simulink model "nonlinsim_bonus"  (R2025a)
settings: Solver=FixedStepAuto  StartTime=0.0  StopTime=100  FixedStep=0.01  RelTol=1e-3
values from neighbouring files (symbols this model uses):
  K_full = zeros(3, 12)    [FP_P9.m]
  u1o = (M + m) * g    (= 5659.275)    [FP_P9.m]    (also in nonlinsim_script.m)
  u2o = 0    [FP_P9.m]    (also in nonlinsim_script.m)
  u3o = 0    [FP_P9.m]    (also in nonlinsim_script.m)
settings Model: Creator=jonl6  LastModifiedBy=kritt
settings SolverCC: AlgebraicLoopSolver=TrustRegion
settings DebuggingCC: UnconnectedInputMsg=warning  UnconnectedOutputMsg=warning  UnconnectedLineMsg=warning
settings ModelReferenceCC: EnableRefExpFcnMdlSchedulingChecks=on
settings RTWCC: GPUComputeCapability=3.5

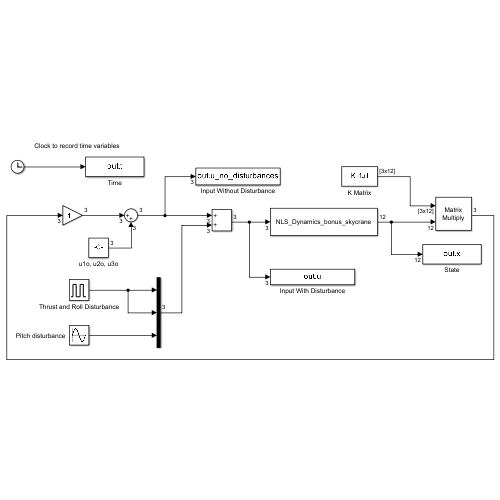
[thumbnail: Simulink's stored preview of the top-level diagram]
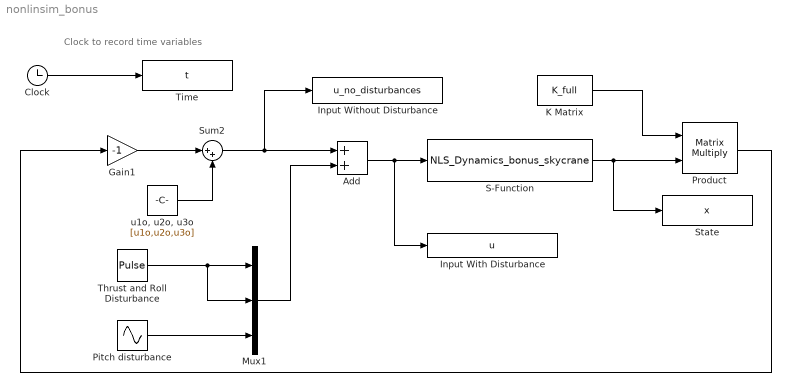
== system nonlinsim_bonus ==
  note: Clock to record time variables
  Add : Sum
  Clock : Clock
  Gain1 : Gain  Gain=-1
  Input With Disturbance : ToWorkspace  VariableName=u  SampleTime=-1
  Input Without Disturbance : ToWorkspace  VariableName=u_no_disturbances  SampleTime=-1
  K Matrix : Constant  Value=K_full
  Mux1 : Mux  Inputs=3
  Pitch disturbance : Sin  Amplitude=1e3  SampleTime=0
  Product : Product  Multiplication=Matrix(*)
  S-Function : S-Function  FunctionName=NLS_Dynamics_bonus_skycrane  Parameters=p  SFunctionDeploymentMode=off  EnableBusSupport=off
  State : ToWorkspace  VariableName=x  SampleTime=-1
  Sum2 : Sum  Inputs=|++
  Thrust and Roll Disturbance : DiscretePulseGenerator  PulseType=Time based  Amplitude=100  Period=100  PulseWidth=10
  Time : ToWorkspace  VariableName=t  SampleTime=-1
  "u1o, u2o, u3o" : Constant  Value=[u1o,u2o,u3o]
  wires:
  Clock/1 -> Time/1
  Mux1/1 -> Add/2
  S-Function/1 -> Product/2, State/1
  K Matrix/1 -> Product/1
  Add/1 -> Input With Disturbance/1, S-Function/1
  Product/1 -> Gain1/1
  Gain1/1 -> Sum2/1
  Pitch disturbance/1 -> Mux1/3
  "u1o, u2o, u3o"/1 -> Sum2/2
  Sum2/1 -> Input Without Disturbance/1, Add/1
  Thrust and Roll Disturbance/1 -> Mux1/2, Mux1/1
